simulink model "bf_bioc_new"  (Simulink 6.0)
settings: Solver=ode15s  StartTime=0.0  StopTime=200  MaxStep=10  MinStep=0.0001  RelTol=1e-3  AbsTol=1e-3
settings Model: LastModifiedBy=cgzkn

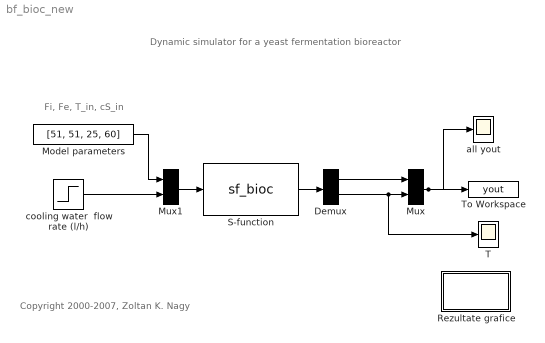
== system bf_bioc_new ==
  note: Dynamic simulator for a yeast fermentation bioreactor
  note: Fi, Fe, T_in, cS_in
  note: Copyright 2000-2007, Zoltan K. Nagy
  Demux : Demux  Outputs=[6 1]
      mask Display: disp('D')
  Model parameters : Constant  Value=[51, 51, 25, 60]
  Mux : Mux  Inputs=[6 1]
      mask Display: disp('M')
  Mux1 : Mux  Inputs=[4 1]
      mask Display: disp('M')
  Rezultate grafice : Subsystem
      settings: OpenFcn=bfgraf
      mask Display: disp('Plot\nresults')
  S-function : S-Function  FunctionName=sf_bioc
      mask Display: disp('BIOREACTOR\nMODEL\ncontinuous')
  T : Scope
      settings: TimeRange=200  YMin=29.5  YMax=32  DataFormat=Array
  To Workspace : ToWorkspace  VariableName=yout  SaveFormat=Array
  all yout : Scope
      settings: TimeRange=200.000000  YMin=-35  YMax=35  DataFormat=Array
  cooling water  flow rate (l/h) : Step  Time=50  Before=18  After=9  SampleTime=0
  wires:
  S-function/1 -> Demux/1
  Demux/1 -> Mux/1
  Demux/2 -> Mux/2, T/1
  Mux/1 -> To Workspace/1, all yout/1
  Model parameters/1 -> Mux1/1
  Mux1/1 -> S-function/1
  cooling water  flow rate (l/h)/1 -> Mux1/2

== system bf_bioc_new/Rezultate grafice ==
